simulink model "shift_register_100_tb"  (R2018b)
settings: Solver=FixedStepAuto  StartTime=0.0  StopTime=100*(15e-9)  FixedStep=15e-9  RelTol=1e-3
libraries: simulink x1
settings Model: Creator=meyer  LastModifiedBy=jason

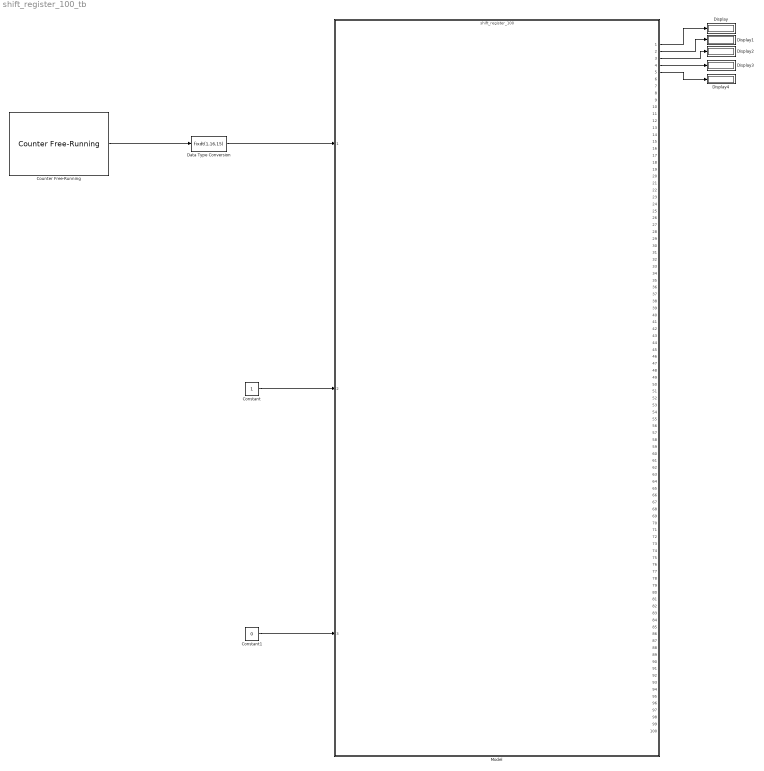
== system shift_register_100_tb ==
  Constant : Constant  OutDataTypeStr=Inherit: Inherit via back propagation  SampleTime=-1
  Constant1 : Constant  Value=0  OutDataTypeStr=Inherit: Inherit via back propagation  SampleTime=-1
  Counter Free-Running : simulink/Sources/Counter Free-Running  NumBits=16  tsamp=-1
  Data Type Conversion : DataTypeConversion  OutDataTypeStr=fixdt(1,16,15)
  Display{,1..4} (5 alike) : Display
  Model : ModelReference  ModelNameDialog=shift_register_100  SimulationMode=Normal  ModelReferenceVersion=1.20
  wires:
  Constant/1 -> Model/2
  Constant1/1 -> Model/3
  Model/1 -> Display/1
  Model/2 -> Display1/1
  Model/3 -> Display2/1
  Model/4 -> Display3/1
  Model/5 -> Display4/1
  Counter Free-Running/1 -> Data Type Conversion/1
  Data Type Conversion/1 -> Model/1
